simulink model "exp_log"  (R2024b)
settings: Solver=VariableStepAuto  StartTime=0.0  StopTime=50  RelTol=1e-3
settings Model: Creator=Botló  LastModifiedBy=Botló

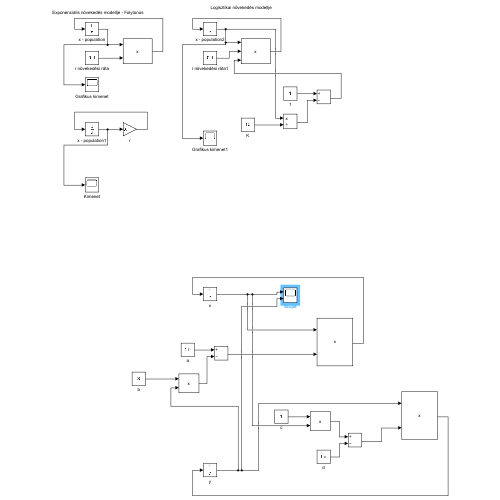
[thumbnail: Simulink's stored preview of the top-level diagram]
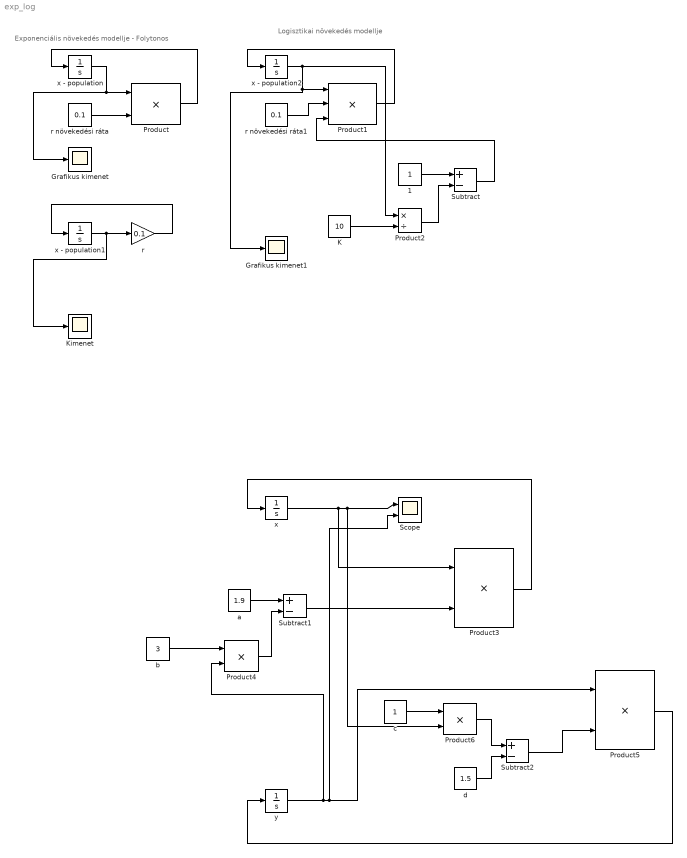
== system exp_log ==
  note: Logisztikai növekedés modellje
  note: Exponenciális növekedés modellje - Folytonos
  1 : Constant
  Grafikus kimenet : Scope
  Grafikus kimenet1 : Scope
  K : Constant  Value=10
  Kimenet : Scope
  Product{,3..6} (5 alike) : Product
  Product1 : Product  Inputs=3
  Product2 : Product  Inputs=*/
  Scope : Scope  NumInputPorts=2
  Subtract : Sum  Inputs=+-
  Subtract1 : Sum  Inputs=+-
  Subtract2 : Sum  Inputs=+-
  a : Constant  Value=1.9
  b : Constant  Value=3
  c : Constant
  d : Constant  Value=1.5
  r : Gain  Gain=0.1
  r növekedési ráta : Constant  Value=0.1
  r növekedési ráta1 : Constant  Value=0.1
  x : Integrator  InitialCondition=0.5
  x - population : Integrator  InitialCondition=1
  x - population1 : Integrator  InitialCondition=50
  x - population2 : Integrator  InitialCondition=1
  y : Integrator  InitialCondition=1.5
  wires:
  r növekedési ráta/1 -> Product/2
  Product/1 -> x - population/1
  x - population/1 -> Grafikus kimenet/1, Product/1
  x - population1/1 -> r/1, Kimenet/1
  r/1 -> x - population1/1
  x - population2/1 -> Product2/1, Grafikus kimenet1/1, Product1/1
  Product1/1 -> x - population2/1
  r növekedési ráta1/1 -> Product1/2
  Subtract/1 -> Product1/3
  1/1 -> Subtract/1
  Product2/1 -> Subtract/2
  K/1 -> Product2/2
  x/1 -> Product3/1, Scope/1, Product6/2
  a/1 -> Subtract1/1
  Product4/1 -> Subtract1/2
  y/1 -> Product4/2, Product5/1, Scope/2
  b/1 -> Product4/1
  Subtract1/1 -> Product3/2
  Product3/1 -> x/1
  Product5/1 -> y/1
  c/1 -> Product6/1
  Product6/1 -> Subtract2/1
  d/1 -> Subtract2/2
  Subtract2/1 -> Product5/2
